simulink model "vienna_pi"  (R2013a)
settings: Solver=ode23tb  StartTime=0.0  StopTime=1  RelTol=1e-3
libraries: powerlib x34, powerlib_extras x1, simulink x1
settings Model: Creator=user  LastModifiedBy=ARJUNpc

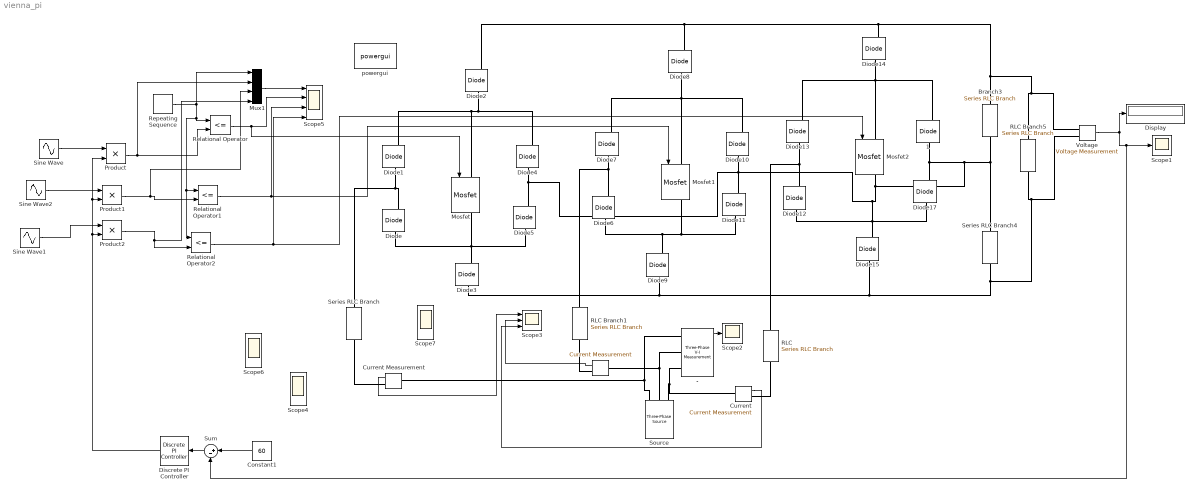
== system vienna_pi ==
  " " : powerlib/Measurements/Current Measurement  PhasorSimulation=off  OutputType=Complex  PSBequivalent=0
  "  Branch3" : powerlib/Elements/Series RLC Branch  LConnTagsString=__new0  RConnTagsString=__new0  BranchType=C  Resistance=1  Inductance=1e-3  SetiL0=off  InitialCurrent=0  Capacitance=5700e-6  Setx0=off  InitialVoltage=0  Measurements=None
  " RLC " : powerlib/Elements/Series RLC Branch  LConnTagsString=__new0  RConnTagsString=__new0  BranchType=L  Resistance=1  Inductance=35e-3  SetiL0=off  InitialCurrent=0  Capacitance=1e-6  Setx0=off  InitialVoltage=0  Measurements=None
  " RLC Branch1" : powerlib/Elements/Series RLC Branch  LConnTagsString=__new0  RConnTagsString=__new0  BranchType=L  Resistance=1  Inductance=35e-3  SetiL0=off  InitialCurrent=0  Capacitance=1e-6  Setx0=off  InitialVoltage=0  Measurements=None
  " RLC Branch5" : powerlib/Elements/Series RLC Branch  LConnTagsString=__new0  RConnTagsString=__new0  BranchType=R  Resistance=10000  Inductance=1e-3  SetiL0=off  InitialCurrent=0  Capacitance=1e-6  Setx0=off  InitialVoltage=0  Measurements=None
  " Source" : powerlib/Electrical Sources/Three-Phase Source  Voltage=12*1.732  PhaseAngle=0  Frequency=50  InternalConnection=Yg  SpecifyImpedance=on  Resistance=0.8929  Inductance=16.58e-3  ShortCircuitLevel=100e6  BaseVoltage=12*1.732  XRratio=7  BusType=swing  Pref=0  Qref=0  Qmin=-inf  Qmax=inf
  "- " : powerlib/Measurements/Three-Phase V-I Measurement  VoltageMeasurement=phase-to-ground  SetLabelV=off  LabelV=Vabc  Vpu=off  VpuLL=off  CurrentMeasurement=yes  SetLabelI=off  LabelI=Iabc  Ipu=off  Pbase=100e6  Vbase=500e3  OutputType=Complex  PhasorSimulation=off  PSBequivalent=0
  1 : powerlib/Power Electronics/Diode  Ron=0.001  Lon=0  Vf=0.8  IC=0  UseSnubber=off  Rs=500  Cs=250e-9  Measurements=on
  Constant1 : Constant  Value=60
  "Current " : powerlib/Measurements/Current Measurement  PhasorSimulation=off  OutputType=Complex  PSBequivalent=0
  Current Measurement : powerlib/Measurements/Current Measurement  PhasorSimulation=off  OutputType=Complex  PSBequivalent=0
  Diode{,1..15,17} (17 alike) : powerlib/Power Electronics/Diode  Ron=0.001  Lon=0  Vf=0.8  IC=0  UseSnubber=off  Rs=500  Cs=250e-9  Measurements=on
  Discrete PI Controller : powerlib_extras/Discrete  Control Blocks/Discrete PI Controller  Kp=0.15  Ki=0.02355  Par_Limits=[1e6 -1e6]  Init=0  Ts=50e-6
  Display : Display
  Mosfet : powerlib/Power Electronics/Mosfet  Ron=0.1  Lon=0  Rd=0.01  Vfd=0  IC=0  Rs=1e5  Cs=inf  Measurements=on
  Mosfet1 : powerlib/Power Electronics/Mosfet  Ron=0.1  Lon=0  Rd=0.01  Vfd=0  IC=0  Rs=1e5  Cs=inf  Measurements=on
  Mosfet2 : powerlib/Power Electronics/Mosfet  Ron=0.1  Lon=0  Rd=0.01  Vfd=0  IC=0  Rs=1e5  Cs=inf  Measurements=on
  Mux1 : Mux
  Product : Product
  Product1 : Product
  Product2 : Product
  Relational Operator : RelationalOperator  Operator=<=  OutDataTypeStr=boolean
  Relational Operator1 : RelationalOperator  Operator=<=  OutDataTypeStr=boolean
  Relational Operator2 : RelationalOperator  Operator=<=  OutDataTypeStr=boolean
  Repeating Sequence : simulink/Sources/Repeating Sequence  rep_seq_t=[0 0.05e-3 0.1e-3 0.15e-3 0.2e-3]  rep_seq_y=[0 1 0 1 0]
  Scope1 : Scope
      settings: YMin=0  YMax=170
  Scope2 : Scope
      settings: YMin=12.454  YMax=12.455  SaveName=ScopeData2
  Scope3 : Scope  NumInputPorts=3
      settings: TimeRange=1  YMin=-0.2~-0.25~-1.75  YMax=1.1~1.75~0.25  SaveName=ScopeData3
  Scope{4..7} (4 alike) : Scope  NumInputPorts=4
      Scope4 settings: YMin=-1~0.95~-5~-5  YMax=1~1.05~5~5
      Scope5 settings: YMin=-1~0.95~-5~-5  YMax=1~1.05~5~5  SaveName=ScopeData5
      Scope6 settings: YMin=-1~0.95~-5~-5  YMax=1~1.05~5~5  SaveName=ScopeData4
      Scope7 settings: YMin=-1~0.95~-5~-5  YMax=1~1.05~5~5  SaveName=ScopeData6
  Series RLC Branch : powerlib/Elements/Series RLC Branch  LConnTagsString=__new0  RConnTagsString=__new0  BranchType=L  Resistance=1  Inductance=35e-3  SetiL0=off  InitialCurrent=0  Capacitance=1e-6  Setx0=off  InitialVoltage=0  Measurements=None
  Series RLC Branch4 : powerlib/Elements/Series RLC Branch  LConnTagsString=__new0  RConnTagsString=__new0  BranchType=C  Resistance=1  Inductance=1e-3  SetiL0=off  InitialCurrent=0  Capacitance=5700e-6  Setx0=off  InitialVoltage=0  Measurements=None
  Sine Wave : Sin  Frequency=100*pi  SampleTime=0
  Sine Wave1 : Sin  Frequency=100*pi  Phase=120*(pi/180)  SampleTime=0
  Sine Wave2 : Sin  Frequency=100*pi  Phase=240*(pi/180)  SampleTime=0
  Sum : Sum  Inputs=|+-
  "Voltage " : powerlib/Measurements/Voltage Measurement  PhasorSimulation=off  OutputType=Complex  PSBequivalent=0
  powergui : powerlib/powergui  Priority=1  SimulationMode=Discrete  SolverType=Tustin  SampleTime=50e-7  frequency=60  SPID=off  DisableSnubberDevices=off  DisableRonSwitches=off  DisableVfSwitches=off  SwTol=0  Interpol=off  DisplayEquations=off  frequencyindice=0  Pbase=100e6  ErrMax=1e-4  Iterations=50  UnitsV=kV  UnitsW=MW  FunctionMessages=off  echomessages=off  HookPort=off  EnableUseOfTLC=off  x0status=blocks  RestoreLinks=warning  ResistiveCurrentMeasurement=off  Frange=[0:2:500]  Ylog=off  Xlog=on  ShowGrid=off  save=off  variable=ZData  ZoomFFT=off  StartTime=0.0  cycles=1  DisplayStyle=1  fundamental=60  FreqAxis=off  MaxFrequency=1000  frequencyindicesteady=1  RmsSteady=1  display=off  Ts=0  methode=off
  wires:
  "Voltage "/1 -> Sum/2, Scope1/1, Display/1
  Current Measurement/1 -> Scope3/1
  " "/1 -> Scope3/2
  "Current "/1 -> Scope3/3
  Repeating Sequence/1 -> Relational Operator2/1, Relational Operator1/1, Relational Operator/1, Mux1/1
  Relational Operator1/1 -> Mosfet1/1, Scope5/3
  Relational Operator2/1 -> Mosfet2/1, Scope5/4
  Relational Operator/1 -> Scope5/2, Mosfet/1
  Mux1/1 -> Scope5/1
  "- "/1 -> Scope2/1
  Constant1/1 -> Sum/1
  Sum/1 -> Discrete PI Controller/1
  Discrete PI Controller/1 -> Product1/2, Product/2, Product2/2
  Sine Wave/1 -> Product/1
  Sine Wave2/1 -> Product1/1
  Sine Wave1/1 -> Product2/1
  Product/1 -> Mux1/2, Relational Operator/2
  Product1/1 -> Mux1/3, Relational Operator1/2
  Product2/1 -> Relational Operator2/2, Mux1/4
  connections:
  Diode1/LConn1 -- Diode/RConn1 -- Series RLC Branch/LConn1
  Diode/LConn1 -- Mosfet/RConn1 -- Diode5/LConn1 -- Diode3/RConn1
  Diode1/RConn1 -- Mosfet/LConn1 -- Diode4/RConn1 -- Diode2/LConn1
  Diode9/RConn1 -- Mosfet1/RConn1 -- Diode11/LConn1 -- Diode6/LConn1
  Diode7/LConn1 -- Diode6/RConn1 -- " RLC Branch1"/LConn1
  Diode12/RConn1 -- " RLC "/LConn1 -- Diode13/LConn1
  "- "/LConn1 -- Current Measurement/LConn1 -- " Source"/RConn1
  "- "/LConn2 -- " Source"/RConn2 -- " "/LConn1
  "- "/LConn3 -- " Source"/RConn3 -- "Current "/LConn1
  Diode15/LConn1 -- Series RLC Branch4/RConn1 -- "Voltage "/LConn2 -- " RLC Branch5"/RConn1 -- Diode3/LConn1 -- Diode9/LConn1
  Diode17/LConn1 -- Mosfet2/RConn1 -- Series RLC Branch4/LConn1 -- "  Branch3"/RConn1 -- Diode17/RConn1 -- 1/LConn1 -- Diode4/LConn1 -- Diode5/RConn1 -- Diode10/LConn1 -- Diode11/RConn1 -- Diode12/LConn1 -- Diode15/RConn1
  1/RConn1 -- Mosfet2/LConn1 -- Diode13/RConn1 -- Diode14/LConn1
  Current Measurement/RConn1 -- Series RLC Branch/RConn1
  "Current "/RConn1 -- " RLC "/RConn1
  " "/RConn1 -- " RLC Branch1"/RConn1
  Diode8/RConn1 -- Diode14/RConn1 -- "  Branch3"/LConn1 -- " RLC Branch5"/LConn1 -- "Voltage "/LConn1 -- Diode2/RConn1
  Diode10/RConn1 -- Mosfet1/LConn1 -- Diode8/LConn1 -- Diode7/RConn1
